simulink model "position_control_z"  (R2023b)
settings: Solver=FixedStepAuto  StartTime=0.0  StopTime=10  RelTol=1e-3  EnableMultiTasking=on
undefined symbols (not defined in the file): DiscIntNeverNeededParam, K, Ts
libraries: cstblocks x2
settings Model: ExtModeTrigDuration=10  Creator=miche  LastModifiedBy=miche
settings OptimizationCC: EnhancedBackFolding=on  PassReuseOutputArgsAs=Individual arguments  ZeroExternalMemoryAtStartup=off  ZeroInternalMemoryAtStartup=off  MaxStackSize=64  OptimizeBlockOrder=speed  DifferentSizesBufferReuse=on  OptimizationCustomize=off  EfficientTunableParamExpr=on
settings DebuggingCC: ParameterTunabilityLossMsg=error
settings HardwareCC: ProdBitPerPointer=32  ProdBitPerSizeT=32  ProdBitPerPtrDiffT=32  ProdLargestAtomicInteger=Long  ProdLargestAtomicFloat=Double  ProdWordSize=32  ProdLongLongMode=on  ProdHWDeviceType=ARM Compatible->ARM Cortex
settings SFSimCC: MATLABDynamicMemAlloc=off
settings RTWCC: Description=Embedded Coder  SystemTargetFile=ert.tlc  HardwareBoard=STM32 Nucleo F401RE  TemplateMakefile=ert_default_tmf  Toolchain=GNU Tools for ARM Embedded Processors  PortableWordSizes=on
settings CodeAppCC: ForceParamTrailComments=on  IgnoreCustomStorageClasses=off  OperatorAnnotations=on  SimulinkDataObjDesc=on  SFDataObjDesc=on  InsertBlockDesc=on
settings ERTTargetCC: ExtModeTransport=3  ExtModeStaticAlloc=on  ExtModeStaticAllocSize=2000  ExtModeMexFile=ext_xcp  ExtModeIntrfLevel=Level2 - Open

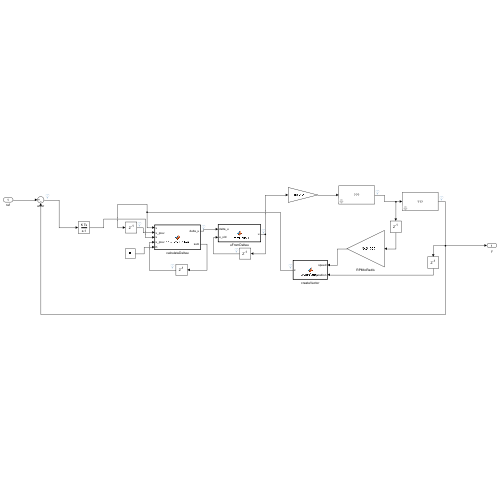
[thumbnail: Simulink's stored preview of the top-level diagram]
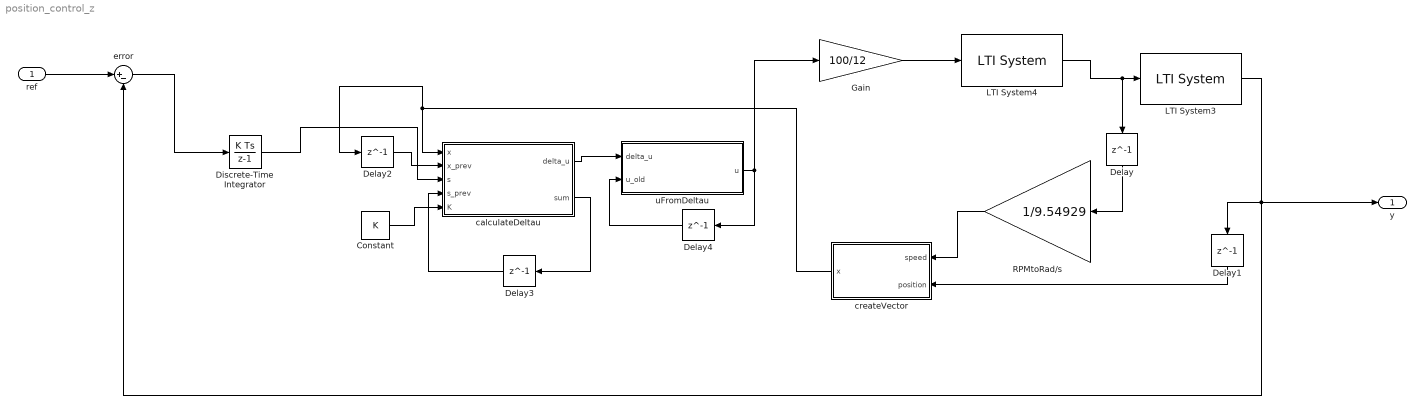
== system position_control_z ==
  ref : Inport  OutDataTypeStr=double  PortDimensions=1  Interpolate=off
  Constant : Constant  Value=K
  Delay : Delay  DelayLength=1
  Delay1 : Delay  DelayLength=1
  Delay2 : Delay  DelayLength=1  InitialCondition=0  SampleTime=Ts
  Delay3 : Delay  DelayLength=1  InitialCondition=0  SampleTime=Ts
  Delay4 : Delay  DelayLength=1  InitialCondition=0  SampleTime=Ts
  Discrete-Time Integrator : DiscreteIntegrator  SampleTime=-1  ICPrevOutput=DiscIntNeverNeededParam  ICPrevScaledInput=DiscIntNeverNeededParam
  Gain : Gain  Gain=100/12
  LTI System3 : cstblocks/LTI System  sys=d_z  IC=[]  PadeOrder=0
  LTI System4 : cstblocks/LTI System  sys=G_z  IC=[]  PadeOrder=0
  RPMtoRad/s : Gain  Gain=1/9.54929
  calculateDeltau : MATLAB Function  TreatAsAtomicUnit=on
  createVector : MATLAB Function  TreatAsAtomicUnit=on
  error : Sum  Inputs=|+-
  uFromDeltau : MATLAB Function  TreatAsAtomicUnit=on
  y : Outport  OutDataTypeStr=double  VectorParamsAs1DForOutWhenUnconnected=off
  wires:
  Gain/1 -> LTI System4/1
  RPMtoRad/s/1 -> createVector/1(speed)
  ref/1 -> error/1
  LTI System3/1 -> error/2, Delay1/1, y/1
  LTI System4/1 -> Delay/1, LTI System3/1
  Delay/1 -> RPMtoRad/s/1
  Delay1/1 -> createVector/2(position)
  error/1 -> Discrete-Time Integrator/1
  calculateDeltau/1(delta_u) -> uFromDeltau/1(delta_u)
  Delay4/1 -> uFromDeltau/2(u_old)
  Delay3/1 -> calculateDeltau/4(s_prev)
  calculateDeltau/2(sum) -> Delay3/1
  Discrete-Time Integrator/1 -> calculateDeltau/3(s)
  createVector/1(x) -> Delay2/1, calculateDeltau/1(x)
  uFromDeltau/1(u) -> Gain/1, Delay4/1
  Constant/1 -> calculateDeltau/5(K)
  Delay2/1 -> calculateDeltau/2(x_prev)

== matlab function position_control_z/calculateDeltau ==
  data: x input; x_prev input; s input; s_prev input; K input; delta_u output; sum output
function [delta_u, sum]= calculateDeltau(x, x_prev, s, s_prev, K)
sum=s;

K1=K(1);
K2=K(2);
K_i=K(3);

delta_x = (x-x_prev);
delta_s = (s-s_prev);

a = -[K1 K2]* delta_x;

b = -K_i*delta_s

delta_u = a+b;

== matlab function position_control_z/uFromDeltau ==
  data: delta_u input; u_old input; u output
function u = uFromDeltau(delta_u, u_old)
    u = u_old+delta_u;
    if u < -12
        u=-12
    end
    if u > 12
        u=12
    end

== matlab function position_control_z/createVector ==
  data: speed input; x output; position input
function x = createVector(speed,position)

x = [speed; position];
